simulink library "csu_lak_linear_accel_kinematics_lib"  (R2014b)
settings: Solver=ode45  SolverMode=SingleTasking  StartTime=0.0  StopTime=10.0  RelTol=1e-3
libraries: util_quat_lib x3, util_common_lib x3, util_info_lib x1
settings Model: Creator=hcannon  LastModifiedBy=mstewart

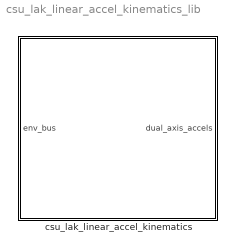
== system csu_lak_linear_accel_kinematics_lib ==
  csu_lak_linear_accel_kinematics : Subsystem  mask{accel_position=[0 0 0], accel_axis_body_frame_1=[0 0 1], accel_axis_body_frame_2=[1 0 0]}
      mask prompts: accel_position "Accelerometer Position in Body Frame"; accel_axis_body_frame_1 "Acceleromter axis 1 direction in body frame"; accel_axis_body_frame_2 "Acceleromter axis 2 direction in body frame"

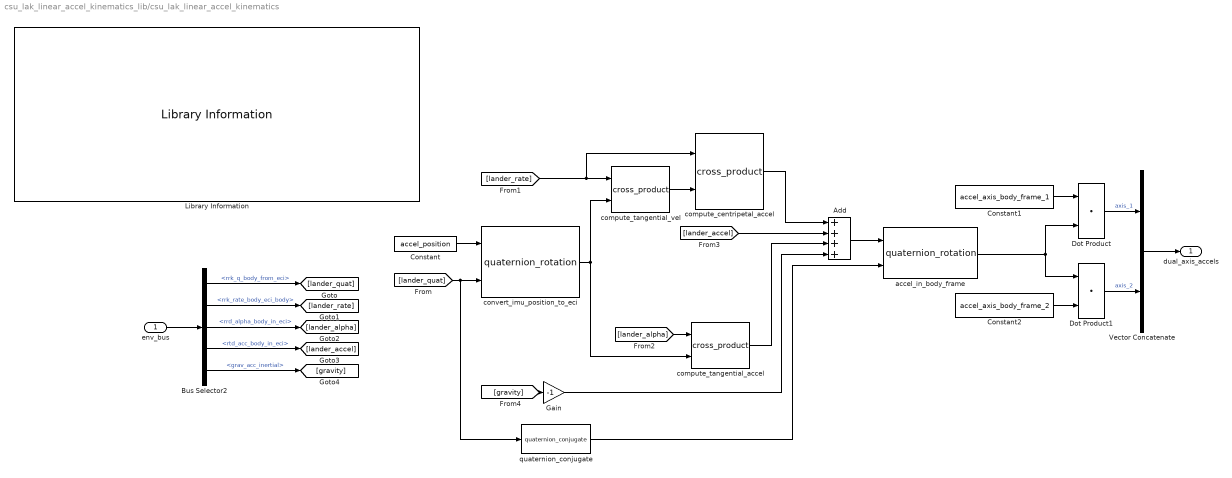
== system csu_lak_linear_accel_kinematics_lib/csu_lak_linear_accel_kinematics ==
  env_bus : Inport
  Add : Sum  Inputs=++++
  Bus Selector2 : BusSelector  OutputSignals=lander_state_bus.rrk_q_body_from_eci,lander_state_bus.rrk_rate_body_eci_body,lander_state_bus.rrd_alpha_body_in_eci,lander_state_bus.rtd_acc_body_in_eci,enf_force_torque_msg.grav_acc_inertial
  Constant : Constant  Value=accel_position
  Constant1 : Constant  Value=accel_axis_body_frame_1  VectorParams1D=off
  Constant2 : Constant  Value=accel_axis_body_frame_2  VectorParams1D=off
  Dot Product : DotProduct  InputSameDT=on  OutDataTypeStr=Inherit: Inherit via internal rule
  Dot Product1 : DotProduct  InputSameDT=on  OutDataTypeStr=Inherit: Inherit via internal rule
  Gain : Gain  Gain=-1
  Library Information : util_info_lib/Library Information  owner='escrane'
  Vector Concatenate : Concatenate
  accel_in_body_frame : util_quat_lib/quaternion_rotation  SystemSampleTime=-1
  compute_centripetal_accel : util_common_lib/cross_product  SystemSampleTime=-1
  compute_tangential_accel : util_common_lib/cross_product  SystemSampleTime=-1
  compute_tangential_vel : util_common_lib/cross_product  SystemSampleTime=-1
  convert_imu_position_to_eci : util_quat_lib/quaternion_rotation  SystemSampleTime=-1
  quaternion_conjugate : util_quat_lib/quaternion_conjugate  SystemSampleTime=-1
  dual_axis_accels : Outport
  wires:
  Constant/1 -> convert_imu_position_to_eci/1
  Constant1/1 -> Dot Product/1
  Add/1 -> accel_in_body_frame/1
  Gain/1 -> Add/4
  [gravity] -> Gain/1
  compute_tangential_accel/1 -> Add/3
  compute_centripetal_accel/1 -> Add/1
  compute_tangential_vel/1 -> compute_centripetal_accel/2
  [lander_rate] -> compute_centripetal_accel/1, compute_tangential_vel/1
  [lander_alpha] -> compute_tangential_accel/1
  convert_imu_position_to_eci/1 -> compute_tangential_vel/2, compute_tangential_accel/2
  [lander_quat] -> convert_imu_position_to_eci/2, quaternion_conjugate/1
  [lander_accel] -> Add/2
  quaternion_conjugate/1 -> accel_in_body_frame/2
  accel_in_body_frame/1 -> Dot Product1/1, Dot Product/2
  Constant2/1 -> Dot Product1/2
  Dot Product/1 -> Vector Concatenate/1  "axis_1"
  Dot Product1/1 -> Vector Concatenate/2  "axis_2"
  Vector Concatenate/1 -> dual_axis_accels/1
  Bus Selector2/5 -> [gravity]  "<grav_acc_inertial>"
  Bus Selector2/4 -> [lander_accel]  "<rtd_acc_body_in_eci>"
  Bus Selector2/3 -> [lander_alpha]  "<rrd_alpha_body_in_eci>"
  Bus Selector2/2 -> [lander_rate]  "<rrk_rate_body_eci_body>"
  Bus Selector2/1 -> [lander_quat]  "<rrk_q_body_from_eci>"
  env_bus/1 -> Bus Selector2/1
